simulink model "Pendulocontrol"  (R2022b)
settings: Solver=VariableStepAuto  StartTime=0.0  StopTime=100  FixedStep=0.01  MaxStep=0.1  MinStep=0.01  RelTol=1e-3
model workspace (MAT data in the model file):
  K = 0.3
  W = 1.25
  k = 0.3
  w = 1.25
  x0 = 0
  y0 = 0
undefined symbols (not defined in the file): sigbuilder_block
settings Model: NumberOfSteps=10  Creator=WINDOWS  LastModifiedBy=WINDOWS
settings DataIOCC: SaveFormat=Array  OutputTimes=tout

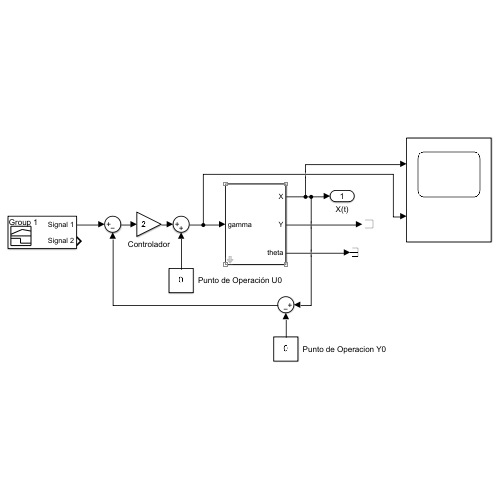
[thumbnail: Simulink's stored preview of the top-level diagram]
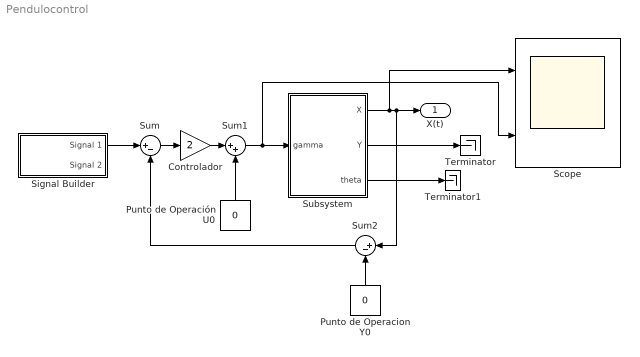
== system Pendulocontrol ==
  Controlador : Gain  Gain=2
  Punto de Operacion Y0 : Constant  Value=0
  Punto de Operación U0 : Constant  Value=0
  Scope : Scope  NumInputPorts=2
  Signal Builder : Subsystem  Tag=STV Subsys  LoadFcn=sigbuilder_block('load',[420.6 113.4 550.8 400.2 ]);  StartFcn=sigbuilder_block('start');  StopFcn=sigbuilder_block('stop');  ClipboardFcn=sigbuilder_block('clipboard');  mask(Sigbuilder block){tuvar=[0:10]}
      mask help: Simulink:masks:SigbuilderBlock_MD
      mask init:
      | if ~strcmp(get_param(bdroot(gcbh),'SimulationStatus'),'stopped') tuvar = sigbuilder_block('maskInit'); end
      settings: CopyFcn=sigbuilder_block('copy');  DeleteFcn=sigbuilder_block('delete');  ModelCloseFcn=sigbuilder_block('modelClose');  PreSaveFcn=sigbuilder_block('preSave');  PauseFcn=sigbuilder_block('pause');  ContinueFcn=sigbuilder_block('continue');  NameChangeFcn=sigbuilder_block('namechange');  OpenFcn=sigbuilder_block('open',[420.6 113.4 550.8 400.2 ]);  CloseFcn=sigbuilder_block('close');
      mask Display: plot(0, 0, 100, 100,[2, 2, 32, 32, 2], [68, 8, 8, 68, 68],[32, 2], [38, 38], [32, 19, 2],[53, 60, 44], [32, 17, 17, 2],[16, 16, 31, 31]);txt = getActiveGroup(gcbh);text(2, 100, txt,'verticalAlignment', 'top');
  Subsystem : Subsystem  mask{k=0.3, w=0, x0=0, y0=0, theta0=0}
  Sum : Sum  Inputs=|+-
  Sum1 : Sum  Inputs=|++
  Sum2 : Sum  Inputs=|+-
  Terminator : Terminator
  Terminator1 : Terminator
  X(t) : Outport
  wires:
  Subsystem/3(theta) -> Terminator1/1
  Punto de Operación U0/1 -> Sum1/2
  Controlador/1 -> Sum1/1
  Sum1/1 -> Scope/2, Subsystem/1(gamma)
  Sum/1 -> Controlador/1
  Punto de Operacion Y0/1 -> Sum2/2
  Sum2/1 -> Sum/2
  Subsystem/1(X) -> Scope/1, X(t)/1, Sum2/1
  Subsystem/2(Y) -> Terminator/1
  Signal Builder/1(Signal 1) -> Sum/1

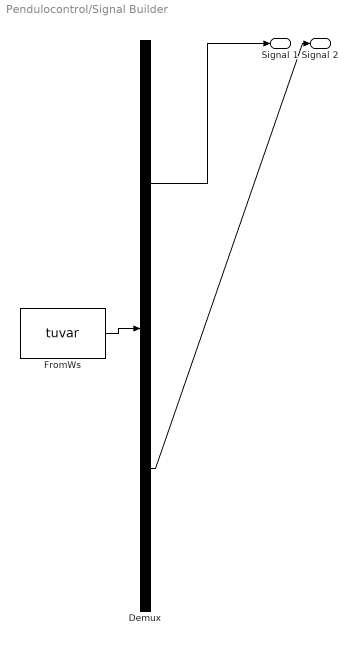
== system Pendulocontrol/Signal Builder ==
  Demux : Demux  Tag=STV Demux  Outputs=2
      settings: DisplayOption=none
  FromWs : FromWorkspace  Tag=STV FromWs  VariableName=tuvar
      SigBuilderData=|
      | common.afterFinalStr = 'Extrapolate'
      | common.sampleTime = 0
      | dataSet.timeRange = [0 100]
      | dataSet.name = 'Group 1'
      | sbobj.Groups.Name = 'Group 1'
      | sbobj.Groups.Signals(1).Name = 'Signal 1'
      | sbobj.Groups.Signals(1).XData = [0 0.2 0.2 50 50 100]
      | sbobj.Groups.Signals(1).YData = [0 0.53 1.005 1 0.5 0]
      | sbobj.Groups.Signals(2).Name = 'Signal 2'
      | sbobj.Groups.Signals(2).XData = [0 50 50 100]
      | sbobj.Groups.Signals(2).YData = [0 0 1 1]
      | sbobj.Groups.TimeRange = [0 100]
  Signal 1 : Outport  Tag=STV Outport
  Signal 2 : Outport  Tag=STV Outport  Port=2
  wires:
  Demux/1 -> Signal 1/1
  FromWs/1 -> Demux/1
  Demux/2 -> Signal 2/1

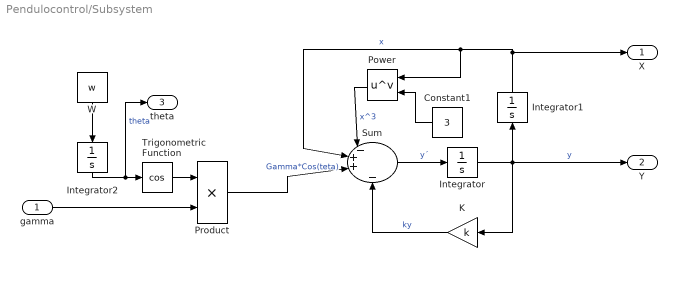
== system Pendulocontrol/Subsystem ==
  gamma : Inport
  Constant1 : Constant  Value=3
  Integrator : Integrator  InitialCondition=y0
  Integrator1 : Integrator  InitialCondition=x0
  Integrator2 : Integrator  InitialCondition=theta0
  K : Gain  Gain=k
  Power : Math  Operator=pow
  Product : Product
  Sum : Sum  Inputs=|-++|-
  Trigonometric Function : Trigonometry  Operator=cos
  W : Constant  Value=w
  X : Outport
  Y : Outport  Port=2
  theta : Outport  Port=3
  wires:
  Trigonometric Function/1 -> Product/1
  Integrator/1 -> Y/1, K/1, Integrator1/1  "y"
  Product/1 -> Sum/3  "Gamma*Cos(teta)"
  Power/1 -> Sum/1  "x^3"
  Constant1/1 -> Power/2
  K/1 -> Sum/4  "ky"
  Integrator1/1 -> Power/1, Sum/2, X/1  "x"
  gamma/1 -> Product/2
  Sum/1 -> Integrator/1  "y´"
  Integrator2/1 -> theta/1, Trigonometric Function/1  "theta"
  W/1 -> Integrator2/1
